simulink model "I_core_control_protected"  (R2023b)
settings: configuration reference "ctrl_tsk_conf" (kept outside this file)
undefined symbols (not defined in the file): ctrl_tsk_st, DC_ff_max, DC_ff_min, hpfratio, prCurrentCtrl
libraries: simulink x3, spsFirstOrderFilterLib x1
settings Model: DataDictionary=fmuGenerationDictionay.sldd  Creator=Veimar  LastModifiedBy=Veimar
settings ConfigSetRef: SourceName=ctrl_tsk_conf

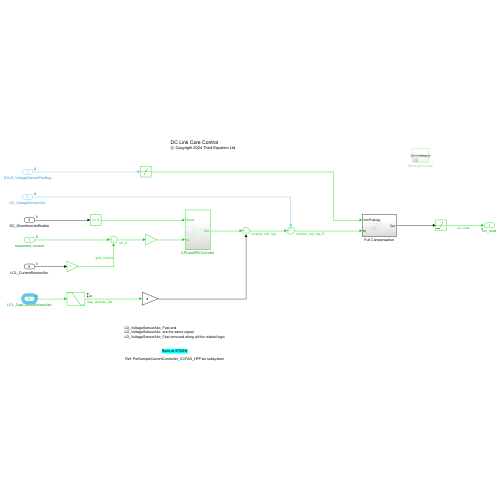
[thumbnail: Simulink's stored preview of the top-level diagram]
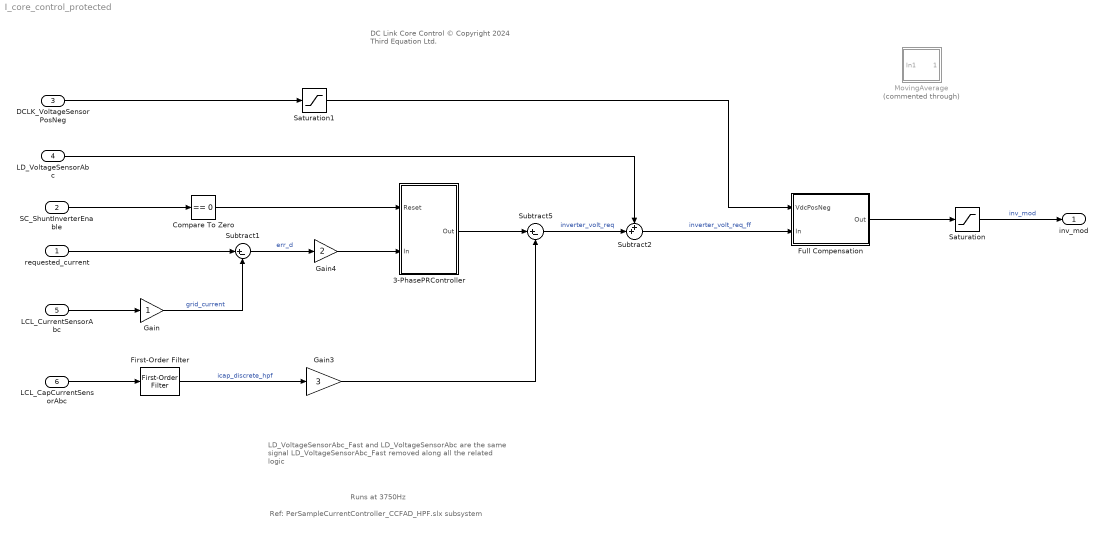
== system I_core_control_protected ==
  note: Runs at 3750Hz
  note: Ref: PerSampleCurrentController_CCFAD_HPF.slx subsystem
  note: DC Link Core Control
      | © Copyright 2024 Third Equation Ltd.
  note: LD_VoltageSensorAbc_Fast and
      | LD_VoltageSensorAbc  are the same signal
      | LD_VoltageSensorAbc_Fast removed along all the related logic
  requested_current : Inport  OutDataTypeStr=single  PortDimensions=3
  SC_ShuntInverterEnable : Inport  Port=2  OutDataTypeStr=boolean  PortDimensions=3
  DCLK_VoltageSensorPosNeg : Inport  Port=3  OutDataTypeStr=single  PortDimensions=2
  LD_VoltageSensorAbc : Inport  Port=4  OutDataTypeStr=single  PortDimensions=3
  LCL_CurrentSensorAbc : Inport  Port=5  OutDataTypeStr=single  PortDimensions=3
  LCL_CapCurrentSensorAbc : Inport  Port=6  OutDataTypeStr=single  PortDimensions=3
  3-PhasePRController : Subsystem
  Compare To Zero : simulink/Logic and Bit Operations/Compare To Zero  relop===  OutDataTypeStr=boolean
  First-Order Filter : spsFirstOrderFilterLib/First-Order Filter  FilterType=Highpass  Tc=ctrl_tsk_st/hpfratio  Ts=ctrl_tsk_st  Initialize=off  Vac_Init=[0, 0, 60]  Vdc_Init=0  PlotResponse=off  FreqRange="[0,  200,  1]"
  Full Compensation : Subsystem
  Gain : Gain
  Gain3 : Gain  Gain=3
  Gain4 : Gain  Gain=2
  MovingAverage : Subsystem  Commented=through
  Saturation : Saturate  UpperLimit=1  LowerLimit=-1  OutDataTypeStr=single
  Saturation1 : Saturate  UpperLimit=DC_ff_max  LowerLimit=DC_ff_min
  Subtract1 : Sum  Inputs=|+-
  Subtract2 : Sum  Inputs=++|
  Subtract5 : Sum  Inputs=|+-
  inv_mod : Outport  OutDataTypeStr=single  PortDimensions=3
  wires:
  DCLK_VoltageSensorPosNeg/1 -> Saturation1/1
  Gain4/1 -> 3-PhasePRController/2(In)
  Compare To Zero/1 -> 3-PhasePRController/1(Reset)
  Full Compensation/1(Out) -> Saturation/1
  Subtract5/1 -> Subtract2/2  "inverter_volt_req"
  Gain/1 -> Subtract1/2  "grid_current"
  requested_current/1 -> Subtract1/1
  Subtract2/1 -> Full Compensation/2(In)  "inverter_volt_req_ff"
  First-Order Filter/1 -> Gain3/1  "icap_discrete_hpf"
  Subtract1/1 -> Gain4/1  "err_d"
  3-PhasePRController/1(Out) -> Subtract5/1
  Saturation/1 -> inv_mod/1  "inv_mod"
  LCL_CurrentSensorAbc/1 -> Gain/1
  LCL_CapCurrentSensorAbc/1 -> First-Order Filter/1
  Gain3/1 -> Subtract5/2
  SC_ShuntInverterEnable/1 -> Compare To Zero/1
  LD_VoltageSensorAbc/1 -> Subtract2/1
  Saturation1/1 -> Full Compensation/1(VdcPosNeg)

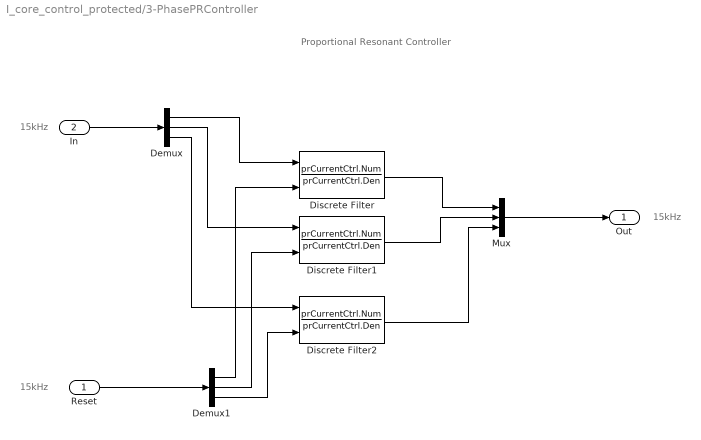
== system I_core_control_protected/3-PhasePRController ==
  note: 15kHz
  note: 15kHz
  note: 15kHz
  note: Proportional Resonant Controller
  Reset : Inport
  In : Inport  Port=2
  Demux : Demux  Outputs=3
  Demux1 : Demux  Outputs=3
  Discrete Filter : DiscreteFilter  Numerator=prCurrentCtrl.Num  Denominator=prCurrentCtrl.Den  ExternalReset=Level
      settings: InputPortMap=u0,r7
  Discrete Filter1 : DiscreteFilter  Numerator=prCurrentCtrl.Num  Denominator=prCurrentCtrl.Den  ExternalReset=Level
      settings: InputPortMap=u0,r7
  Discrete Filter2 : DiscreteFilter  Numerator=prCurrentCtrl.Num  Denominator=prCurrentCtrl.Den  ExternalReset=Level
      settings: InputPortMap=u0,r7
  Mux : Mux  Inputs=3
  Out : Outport
  wires:
  Reset/1 -> Demux1/1
  In/1 -> Demux/1
  Demux1/1 -> Discrete Filter/2
  Demux1/2 -> Discrete Filter1/2
  Demux1/3 -> Discrete Filter2/2
  Demux/1 -> Discrete Filter/1
  Demux/2 -> Discrete Filter1/1
  Demux/3 -> Discrete Filter2/1
  Discrete Filter/1 -> Mux/1
  Discrete Filter1/1 -> Mux/2
  Discrete Filter2/1 -> Mux/3
  Mux/1 -> Out/1

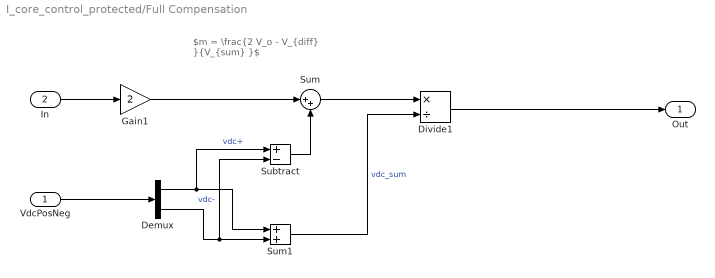
== system I_core_control_protected/Full Compensation ==
  note: $m = \frac{2 V_o - V_{diff} }{V_{sum} }$
  VdcPosNeg : Inport
  In : Inport  Port=2
  Demux : Demux  Outputs=2
  Divide1 : Product  Inputs=*/  OutDataTypeStr=single
  Gain1 : Gain  Gain=2
  Subtract : Sum  Inputs=+-
  Sum : Sum  Inputs=|++
  Sum1 : Sum
  Out : Outport
  wires:
  Divide1/1 -> Out/1
  Gain1/1 -> Sum/1
  VdcPosNeg/1 -> Demux/1
  Sum/1 -> Divide1/1
  Demux/1 -> Sum1/1, Subtract/1  "vdc+"
  Sum1/1 -> Divide1/2  "vdc_sum"
  Demux/2 -> Sum1/2, Subtract/2  "vdc-"
  In/1 -> Gain1/1
  Subtract/1 -> Sum/2

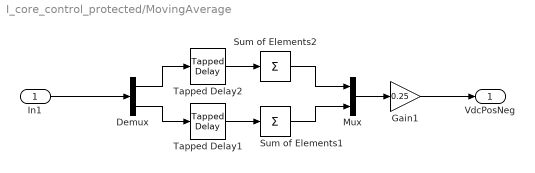
== system I_core_control_protected/MovingAverage ==
  In1 : Inport
  Demux : Demux  Outputs=2
  Gain1 : Gain  Gain=0.25
  Mux : Mux  Inputs=2
  Sum of Elements1 : Sum  Inputs=+
  Sum of Elements2 : Sum  Inputs=+
  Tapped Delay1 : simulink/Discrete/Tapped Delay  vinit=0.0  samptime=-1  NumDelays=3  DelayOrder=Oldest  includeCurrent=on
  Tapped Delay2 : simulink/Discrete/Tapped Delay  vinit=0.0  samptime=-1  NumDelays=3  DelayOrder=Oldest  includeCurrent=on
  VdcPosNeg : Outport
  wires:
  In1/1 -> Demux/1
  Demux/1 -> Tapped Delay2/1
  Tapped Delay2/1 -> Sum of Elements2/1
  Demux/2 -> Tapped Delay1/1
  Gain1/1 -> VdcPosNeg/1
  Sum of Elements2/1 -> Mux/1
  Mux/1 -> Gain1/1
  Tapped Delay1/1 -> Sum of Elements1/1
  Sum of Elements1/1 -> Mux/2
